simulink subsystem "Gear"  (R2023a)
settings: Solver=VariableStepAuto  StartTime=0.0  StopTime=10.0  RelTol=1e-3
values from neighbouring files (symbols this model uses):
  i = 12    [init.m]
  J_screw = 0.006    [init.m]
settings Model: Creator=ycheb  LastModifiedBy=ycheb

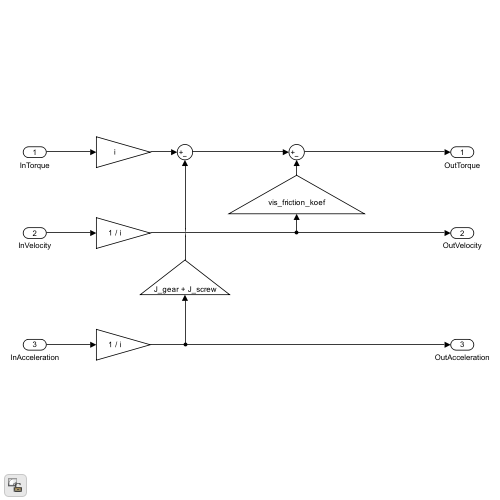
[thumbnail: Simulink's stored preview of the top-level diagram]
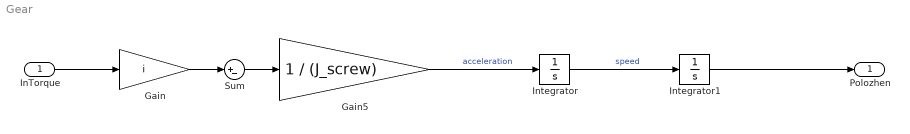
== system Gear ==
  InTorque : Inport
  Gain : Gain  Gain=i
  Gain5 : Gain  Gain=1 / (J_screw)
  Integrator : Integrator
  Integrator1 : Integrator
  Sum : Sum  Inputs=|+-
  Polozhen : Outport
  wires:
  Sum/1 -> Gain5/1
  InTorque/1 -> Gain/1
  Gain/1 -> Sum/1
  Integrator/1 -> Integrator1/1  "speed"
  Integrator1/1 -> Polozhen/1
  Gain5/1 -> Integrator/1  "acceleration"
